simulink model "mCopyParam"  (Simulink 8.0)
settings: Solver=ode45  StartTime=0.0  StopTime=10.0  RelTol=1e-3
settings Model: FPTRunName=Active  Creator=hungdang  LastModifiedBy=hungdang
settings DataIOCC: SignalLoggingSaveFormat=ModelDataLogs
settings OptimizationCC: InlineParams=on
settings DebuggingCC: FcnCallInpInsideContextMsg=Enable All
settings GRTTargetCC: CombineOutputUpdateFcns=off  GRTInterface=on

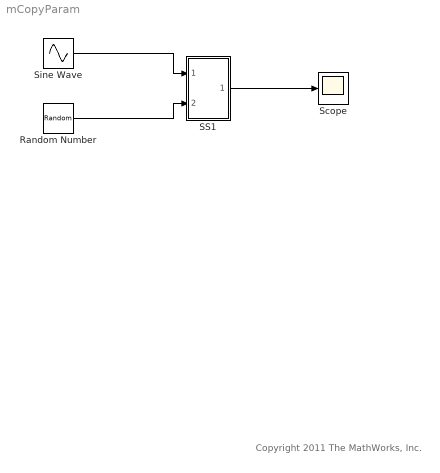
== system mCopyParam ==
  note: Copyright 2011 The MathWorks, Inc.
  Random Number : RandomNumber  SampleTime=0.1
  SS1 : Subsystem  RequirementInfo={'linktype_rmi_url' 'mathworks.com' '' 'true' 'MathWorks' '' ; 'other' 'requirements.txt' '' 'true' 'An external text file' '' } %GIDa_f14b8f86_de21_4f69_a62b_9cfe1636c3f7  TreatAsAtomicUnit=on
      settings: MinAlgLoopOccurrences=on
  Scope : Scope
  Sine Wave : Sin  SampleTime=0
  wires:
  Random Number/1 -> SS1/2(In2)
  Sine Wave/1 -> SS1/1(In1)
  SS1/1(Out1) -> Scope/1

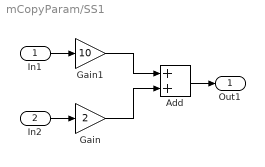
== system mCopyParam/SS1 ==
  In1 : Inport
  In2 : Inport  Port=2
  Add : Sum
  Gain : Gain  Gain=2
  Gain1 : Gain  Gain=10
  Out1 : Outport
  wires:
  Gain1/1 -> Add/1
  Gain/1 -> Add/2
  In1/1 -> Gain1/1
  Add/1 -> Out1/1
  In2/1 -> Gain/1
